simulink model "simulation_gripen_lqg"  (R2021a)
settings: Solver=ode15s  StartTime=0.0  StopTime=200  RelTol=1e-3  EnableMultiTasking=on
values from neighbouring files (symbols this model uses):
  A = [-0.292 -0.152 0.0364 0 0 0 0 8.13 -2.54 -0.0678 1 0 ... (49 elements, 7x7)]    [Gripendata.mat]
  B = [0 -31.7 0 0 0 20 0 -2.15 0.0274 1.48 0 0 ... (14 elements, 7x2)]    [Gripendata.mat]
  C = [0 0 0 0 0 0 1 0 0 1 0 0 ... (14 elements, 2x7)]    [Gripendata.mat]
  D = [0  0; 0  0]    [Gripendata.mat]
  x0 = [5 0.00174532925199 0.00174532925199 0.0872664625997 0.0872664625997 0 0]    [Gripendata.mat]
undefined symbols (not defined in the file or in its folder): A_kf, B_kf, C_kf, D_kf, Klq_eta, Klq_x
settings Model: Creator=scattolini  LastModifiedBy=fabio
settings SolverCC: AlgebraicLoopSolver=TrustRegion
settings DataIOCC: LimitDataPoints=on  SaveFormat=Array  SignalLoggingSaveFormat=ModelDataLogs  ReturnWorkspaceOutputs=off
settings OptimizationCC: ExpressionDepthLimit=2147483647  InitFltsAndDblsToZero=on  LifeSpan=inf
settings DebuggingCC: SaveWithParameterizedLinksMsg=none  UnderspecifiedInitializationDetection=Classic  MergeDetectMultiDrivingBlocksExec=none  SignalResolutionControl=TryResolveAllWithWarning  SolverPrmCheckMsg=warning  MultiTaskDSMMsg=warning  MultiTaskCondExecSysMsg=none  FcnCallInpInsideContextMsg=warning  StateNameClashWarn=warning  SFUnexpectedBacktrackingDiag=warning  SFNoUnconditionalDefaultTransitionDiag=warning  SFExecutionAtInitializationDiag=none  SFMachineParentedDataDiag=warning  ArithmeticOperatorsInVariantConditions=warning
settings HardwareCC: ProdBitPerPointer=32  ProdBitPerSizeT=32  ProdBitPerPtrDiffT=32  ProdLargestAtomicFloat=None  ProdIntDivRoundTo=Undefined  ProdEndianess=Unspecified  ProdWordSize=32  ProdHWDeviceType=32-bit Generic
settings ModelReferenceCC: PropagateSignalLabelsOutOfModel=off
settings SFSimCC: SimUseLocalCustomCode=off  CustomCodeUndefinedFunction=UseInterfaceOnly
settings RTWCC: RTWUseLocalCustomCode=off
settings CodeAppCC: StateflowObjectComments=on
settings GRTTargetCC: TargetFcnLib=ansi_tfl_tmw.mat  TargetLangStandard=C89/C90 (ANSI)  CombineOutputUpdateFcns=off  GRTInterface=on
settings ConfigComp: CovMetricSettings=dw  CovSaveCumulativeToWorkspaceVar=on  CovSaveSingleToWorkspaceVar=on  CovExternalEMLEnable=off

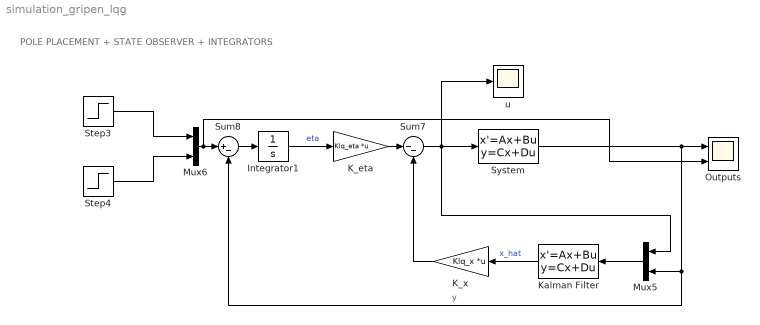
== system simulation_gripen_lqg ==
  note: POLE PLACEMENT + STATE OBSERVER + INTEGRATORS
  Integrator1 : Integrator
  K_eta : Gain  Gain=Klq_eta  Multiplication=Matrix(K*u) (u vector)
  K_x : Gain  Gain=Klq_x  Multiplication=Matrix(K*u) (u vector)
  Kalman Filter : StateSpace  A=A_kf  B=B_kf  C=C_kf  D=D_kf  InitialCondition=0
  Mux5 : Mux  Inputs=2
  Mux6 : Mux  Inputs=2
  Outputs : Scope  NumInputPorts=2
  Step3 : Step  Time=100  After=1.04  SampleTime=0
  Step4 : Step  Time=150  After=-0.52  SampleTime=0
  Sum7 : Sum  Inputs=|--
  Sum8 : Sum  Inputs=|+-
  System : StateSpace  A=A  B=B  C=C  D=D  InitialCondition=x0
  u : Scope
  wires:
  K_x/1 -> Sum7/2
  Mux5/1 -> Kalman Filter/1
  System/1 -> Outputs/1, Mux5/2, Sum8/2  "y"
  Kalman Filter/1 -> K_x/1  "x_hat"
  K_eta/1 -> Sum7/1
  Sum7/1 -> u/1, Mux5/1, System/1
  Integrator1/1 -> K_eta/1  "eta"
  Sum8/1 -> Integrator1/1
  Mux6/1 -> Outputs/2, Sum8/1
  Step3/1 -> Mux6/1
  Step4/1 -> Mux6/2
